simulink model "HA_MPPT_v3"  (R2015a)
settings: Solver=FixedStepDiscrete  StartTime=0  StopTime=86400  FixedStep=0.1  RelTol=1e-3
settings Model: Creator=moury  LastModifiedBy=moury
settings DataIOCC: SignalLogging=off

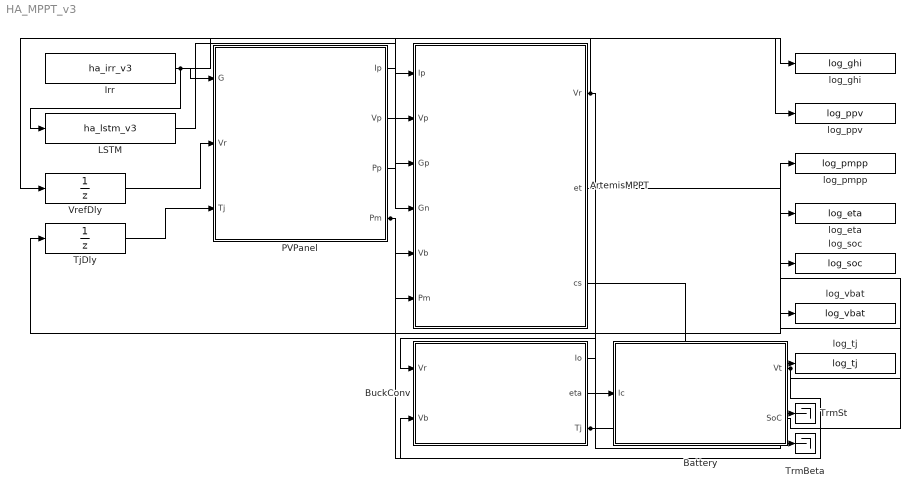
== system HA_MPPT_v3 ==
  ArtemisMPPT : Subsystem
  Battery : Subsystem
  BuckConv : Subsystem
  Irr : S-Function  FunctionName=ha_irr_v3
  LSTM : S-Function  FunctionName=ha_lstm_v3
  PVPanel : Subsystem
  TjDly : UnitDelay  InitialCondition=40  SampleTime=0.1
  TrmBeta : Terminator
  TrmSt : Terminator
  VrefDly : UnitDelay  InitialCondition=17.8  SampleTime=0.1
  log_eta : ToWorkspace  VariableName=log_eta
  log_ghi : ToWorkspace  VariableName=log_ghi
  log_pmpp : ToWorkspace  VariableName=log_pmpp
  log_ppv : ToWorkspace  VariableName=log_ppv
  log_soc : ToWorkspace  VariableName=log_soc
  log_tj : ToWorkspace  VariableName=log_tj
  log_vbat : ToWorkspace  VariableName=log_vbat
  wires:
  Irr/1 -> LSTM/1, PVPanel/1(G), ArtemisMPPT/4(Gn), log_ghi/1
  VrefDly/1 -> PVPanel/2(Vr)
  TjDly/1 -> PVPanel/3(Tj)
  PVPanel/1(Ip) -> ArtemisMPPT/1(Ip)
  PVPanel/2(Vp) -> ArtemisMPPT/2(Vp)
  LSTM/1 -> ArtemisMPPT/3(Gp)
  PVPanel/4(Pm) -> ArtemisMPPT/6(Pm), log_pmpp/1
  ArtemisMPPT/1(Vr) -> VrefDly/1, BuckConv/1(Vr)
  Battery/1(Vt) -> ArtemisMPPT/5(Vb), BuckConv/2(Vb), log_vbat/1
  BuckConv/1(Io) -> Battery/1(Ic)
  BuckConv/3(Tj) -> TjDly/1, log_tj/1
  BuckConv/2(eta) -> TrmBeta/1
  ArtemisMPPT/3(cs) -> TrmSt/1
  PVPanel/3(Pp) -> log_ppv/1
  ArtemisMPPT/2(et) -> log_eta/1
  Battery/2(SoC) -> log_soc/1

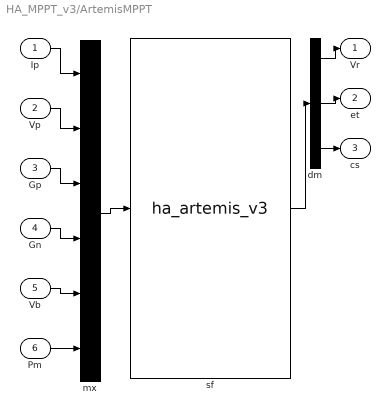
== system HA_MPPT_v3/ArtemisMPPT ==
  Ip : Inport
  Vp : Inport  Port=2
  Gp : Inport  Port=3
  Gn : Inport  Port=4
  Vb : Inport  Port=5
  Pm : Inport  Port=6
  dm : Demux  Outputs=3
  mx : Mux  Inputs=6
  sf : S-Function  FunctionName=ha_artemis_v3
  Vr : Outport
  et : Outport  Port=2
  cs : Outport  Port=3
  wires:
  Ip/1 -> mx/1
  Vp/1 -> mx/2
  Gp/1 -> mx/3
  Gn/1 -> mx/4
  Vb/1 -> mx/5
  Pm/1 -> mx/6
  mx/1 -> sf/1
  sf/1 -> dm/1
  dm/1 -> Vr/1
  dm/2 -> et/1
  dm/3 -> cs/1

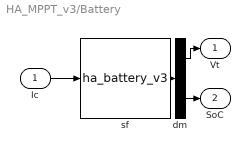
== system HA_MPPT_v3/Battery ==
  Ic : Inport
  dm : Demux  Outputs=2
  sf : S-Function  FunctionName=ha_battery_v3
  Vt : Outport
  SoC : Outport  Port=2
  wires:
  Ic/1 -> sf/1
  sf/1 -> dm/1
  dm/1 -> Vt/1
  dm/2 -> SoC/1

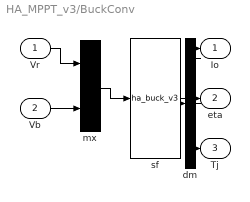
== system HA_MPPT_v3/BuckConv ==
  Vr : Inport
  Vb : Inport  Port=2
  dm : Demux  Outputs=3
  mx : Mux  Inputs=2
  sf : S-Function  FunctionName=ha_buck_v3
  Io : Outport
  eta : Outport  Port=2
  Tj : Outport  Port=3
  wires:
  Vr/1 -> mx/1
  Vb/1 -> mx/2
  mx/1 -> sf/1
  sf/1 -> dm/1
  dm/1 -> Io/1
  dm/2 -> eta/1
  dm/3 -> Tj/1

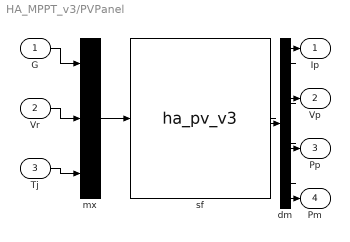
== system HA_MPPT_v3/PVPanel ==
  G : Inport
  Vr : Inport  Port=2
  Tj : Inport  Port=3
  dm : Demux
  mx : Mux  Inputs=3
  sf : S-Function  FunctionName=ha_pv_v3
  Ip : Outport
  Vp : Outport  Port=2
  Pp : Outport  Port=3
  Pm : Outport  Port=4
  wires:
  G/1 -> mx/1
  Vr/1 -> mx/2
  Tj/1 -> mx/3
  mx/1 -> sf/1
  sf/1 -> dm/1
  dm/1 -> Ip/1
  dm/2 -> Vp/1
  dm/3 -> Pp/1
  dm/4 -> Pm/1
